simulink model "Reference_Simulink_Model"  (R2024a)
settings: Solver=VariableStepAuto  StartTime=0.0  StopTime=2800  RelTol=1e-3
undefined symbols (not defined in the file or in its folder): Amplitude_Wave_Lake, Amplitude_Wind_Lake, Factor_Wave_1, Factor_Wave_2, Frequency_Wave_Lake, Frequency_Wind_Lake, Gain_Derivative_Controller, Gain_Integral_Controller, Gain_Proportional_Controller, Gain_Wind, Position_Initial_X, Position_Initial_Y, Static_Gain_Waves, Time_Constant_Wind, Velocity_Ship_Mean, Waypoints
libraries: cstblocks x2, simulink x2
settings Model: Creator=gerar  LastModifiedBy=gerar

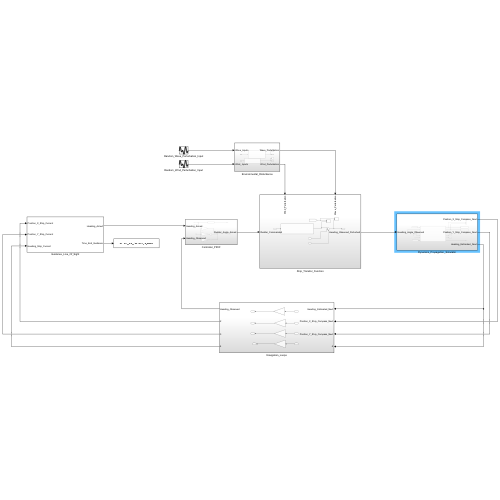
[thumbnail: Simulink's stored preview of the top-level diagram]
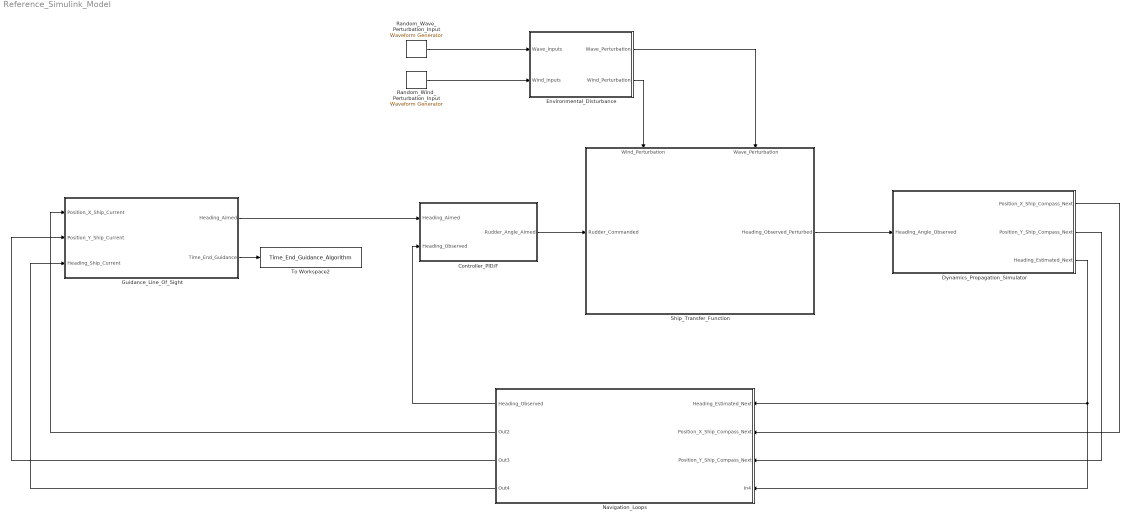
== system Reference_Simulink_Model ==
  Controller_PID/F : Subsystem
  Dynamics_Propagation_Simulator : Subsystem
  Environmental_Disturbance : Subsystem
  Guidance_Line_Of_Sight : Subsystem
  Navigation_Loops : Subsystem
  Random_Wave_Perturbation_Input : simulink/Sources/Waveform Generator  OutMin=[]  OutMax=[]  OutDataTypeStr=double  SelectedSignal=1  Signals=sin(Amplitude_Wave_Lake, Frequency_Wave_Lake, 1)  BlockNames=MultiportSwitch_4566f8e7d9dc4b1  SampleTime=0.1
  Random_Wind_Perturbation_Input : simulink/Sources/Waveform Generator  OutMin=[]  OutMax=[]  OutDataTypeStr=double  SelectedSignal=1  Signals=sin(Amplitude_Wind_Lake, Frequency_Wind_Lake, 1)  BlockNames=MultiportSwitch_bec1be775c304e8  SampleTime=0.1
  Ship_Transfer_Function : Subsystem
      settings: PortSchema="{\"entries\":[{\"content\":{\"sides\":[{\"content\":{\"connectorIds\":[\"In1\"]},\"type\":\"ConnectorPlacement.EquallySpacedRectSide\",\"uuid\":\"39a47681-8a87-4f22-9e16-0ead526089e0\"},{\"content\":{\"connectorIds\":[\"Out1\"],\"side\":\"RIGHT\"},\"type\":\"ConnectorPlacement.EquallySpacedRectSide\",\"uuid\":\"e7d068dc-643f-44db-a553-0a54b66f6b70\"},{\"content\":{\"connectorIds\":[\"In2\",\"In3\"],\"side\":\"TOP\"},\"type\":\"ConnectorPlacement.EquallySpacedRectSide\",\"uuid\":\"f984f23d-1b96-40dd-a354-9bced51babaa\"}]},\"type\":\"ConnectorPlacement.EquallySpacedConnector\",\"uuid\":\"30082198-c592-4bfc-a5f8-ae0235b1924b\"}],\"packageUris\":[\"http://schema.mathworks.com/mf0/Connector/R2020b\"],\"version\":\"1.0\"}"
  To Workspace2 : ToWorkspace  VariableName=Time_End_Guidance_Algorithm  SaveFormat=Timeseries  SampleTime=-1
  wires:
  Guidance_Line_Of_Sight/1(Heading_Aimed) -> Controller_PID/F/1(Heading_Aimed)
  Controller_PID/F/1(Rudder_Angle_Aimed) -> Ship_Transfer_Function/1(Rudder_Commanded)
  Guidance_Line_Of_Sight/2(Time_End_Guidance) -> To Workspace2/1
  Random_Wave_Perturbation_Input/1 -> Environmental_Disturbance/1(Wave_Inputs)
  Random_Wind_Perturbation_Input/1 -> Environmental_Disturbance/2(Wind_Inputs)
  Environmental_Disturbance/1(Wave_Perturbation) -> Ship_Transfer_Function/3(Wave_Perturbation)
  Environmental_Disturbance/2(Wind_Perturbation) -> Ship_Transfer_Function/2(Wind_Perturbation)
  Navigation_Loops/1(Heading_Observed) -> Controller_PID/F/2(Heading_Observed)
  Ship_Transfer_Function/1(Heading_Observed_Perturbed) -> Dynamics_Propagation_Simulator/1(Heading_Angle_Observed)
  Dynamics_Propagation_Simulator/3(Heading_Estimated_Next) -> Navigation_Loops/4(In4), Navigation_Loops/1(Heading_Estimated_Next)
  Dynamics_Propagation_Simulator/1(Position_X_Ship_Compass_Next) -> Navigation_Loops/2(Position_X_Ship_Compass_Next)
  Navigation_Loops/2(Out2) -> Guidance_Line_Of_Sight/1(Position_X_Ship_Current)
  Dynamics_Propagation_Simulator/2(Position_Y_Ship_Compass_Next) -> Navigation_Loops/3(Position_Y_Ship_Compass_Next)
  Navigation_Loops/3(Out3) -> Guidance_Line_Of_Sight/2(Position_Y_Ship_Current)
  Navigation_Loops/4(Out4) -> Guidance_Line_Of_Sight/3(Heading_Ship_Current)

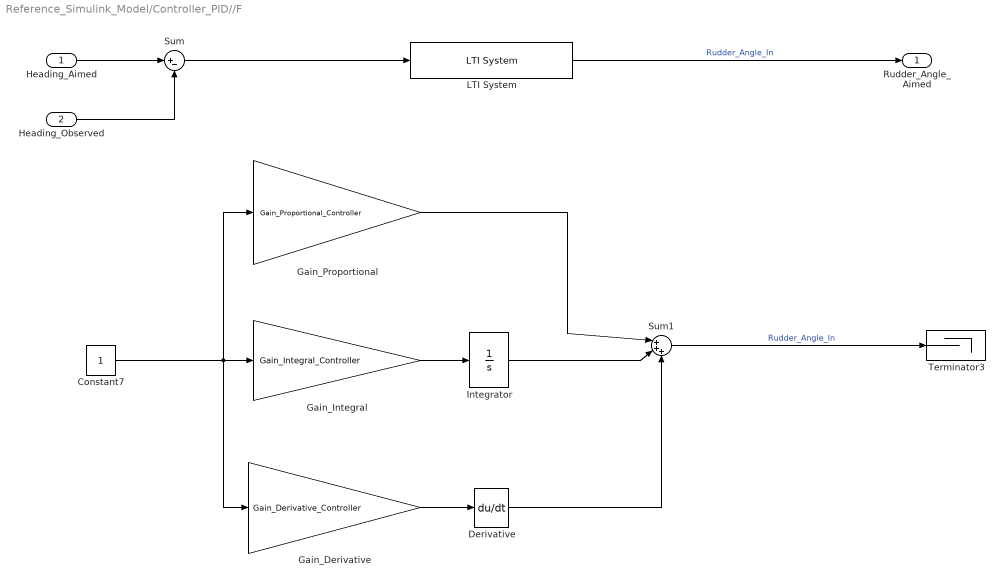
== system Reference_Simulink_Model/Controller_PID//F ==
  Heading_Aimed : Inport
  Heading_Observed : Inport  Port=2
  Constant7 : Constant
  Derivative : Derivative
  Gain_Derivative : Gain  Gain=Gain_Derivative_Controller
  Gain_Integral : Gain  Gain=Gain_Integral_Controller
  Gain_Proportional : Gain  Gain=Gain_Proportional_Controller
  Integrator : Integrator
  LTI System : cstblocks/LTI System  sys=Controller_PIDF  IC=[]  PadeOrder=0
  Sum : Sum  Inputs=|+-
  Sum1 : Sum  Inputs=|+++
  Terminator3 : Terminator
  Rudder_Angle_Aimed : Outport
  wires:
  Heading_Aimed/1 -> Sum/1
  Heading_Observed/1 -> Sum/2
  Sum1/1 -> Terminator3/1  "Rudder_Angle_In"
  Gain_Proportional/1 -> Sum1/1
  Integrator/1 -> Sum1/2
  Gain_Integral/1 -> Integrator/1
  Constant7/1 -> Gain_Proportional/1, Gain_Integral/1, Gain_Derivative/1
  Gain_Derivative/1 -> Derivative/1
  Derivative/1 -> Sum1/3
  Sum/1 -> LTI System/1
  LTI System/1 -> Rudder_Angle_Aimed/1  "Rudder_Angle_In"

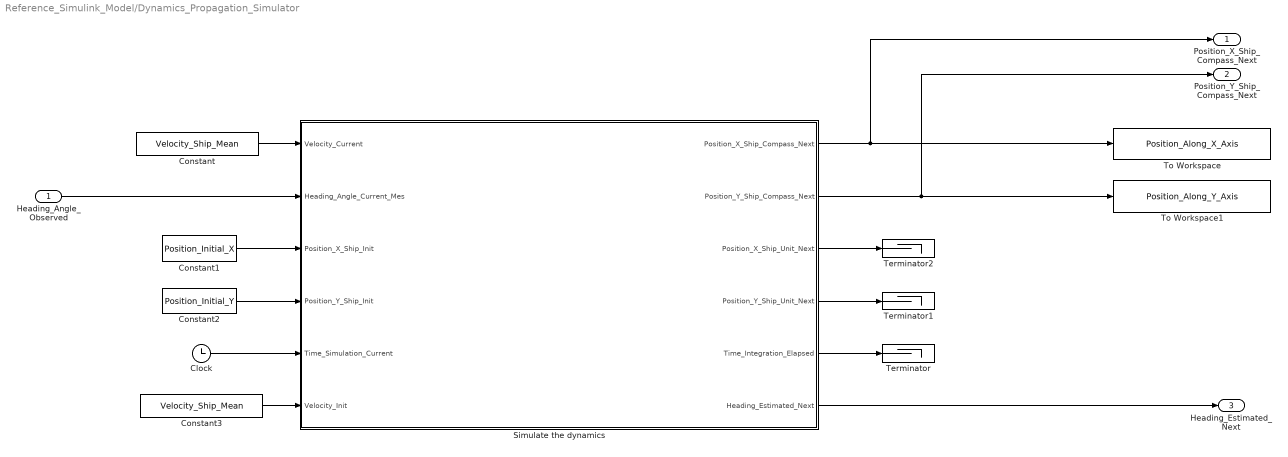
== system Reference_Simulink_Model/Dynamics_Propagation_Simulator ==
  Heading_Angle_Observed : Inport
  Clock : Clock
  Constant : Constant  Value=Velocity_Ship_Mean
  Constant1 : Constant  Value=Position_Initial_X
  Constant2 : Constant  Value=Position_Initial_Y
  Constant3 : Constant  Value=Velocity_Ship_Mean
  Simulate the dynamics : MATLAB Function  TreatAsAtomicUnit=on
  Terminator : Terminator
  Terminator1 : Terminator
  Terminator2 : Terminator
  To Workspace : ToWorkspace  VariableName=Position_Along_X_Axis  SaveFormat=Timeseries  SampleTime=-1
  To Workspace1 : ToWorkspace  VariableName=Position_Along_Y_Axis  SaveFormat=Timeseries  SampleTime=-1
  Position_X_Ship_Compass_Next : Outport
  Position_Y_Ship_Compass_Next : Outport  Port=2
  Heading_Estimated_Next : Outport  Port=3
  wires:
  Simulate the dynamics/1(Position_X_Ship_Compass_Next) -> Position_X_Ship_Compass_Next/1, To Workspace/1
  Heading_Angle_Observed/1 -> Simulate the dynamics/2(Heading_Angle_Current_Mes)
  Simulate the dynamics/5(Time_Integration_Elapsed) -> Terminator/1
  Simulate the dynamics/4(Position_Y_Ship_Unit_Next) -> Terminator1/1
  Constant1/1 -> Simulate the dynamics/3(Position_X_Ship_Init)
  Constant/1 -> Simulate the dynamics/1(Velocity_Current)
  Simulate the dynamics/2(Position_Y_Ship_Compass_Next) -> Position_Y_Ship_Compass_Next/1, To Workspace1/1
  Simulate the dynamics/3(Position_X_Ship_Unit_Next) -> Terminator2/1
  Constant2/1 -> Simulate the dynamics/4(Position_Y_Ship_Init)
  Clock/1 -> Simulate the dynamics/5(Time_Simulation_Current)
  Simulate the dynamics/6(Heading_Estimated_Next) -> Heading_Estimated_Next/1
  Constant3/1 -> Simulate the dynamics/6(Velocity_Init)

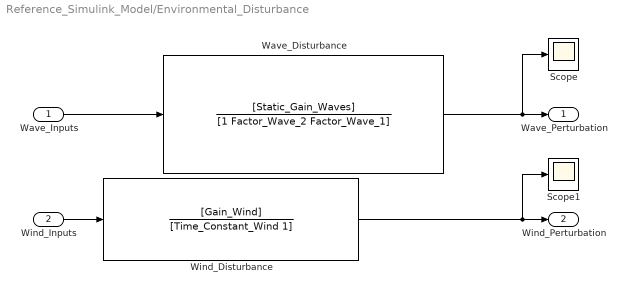
== system Reference_Simulink_Model/Environmental_Disturbance ==
  Wave_Inputs : Inport
  Wind_Inputs : Inport  Port=2
  Scope : Scope
  Scope1 : Scope
  Wave_Disturbance : TransferFcn  Numerator=[Static_Gain_Waves]  Denominator=[1 Factor_Wave_2 Factor_Wave_1]
  Wind_Disturbance : TransferFcn  Numerator=[Gain_Wind]  Denominator=[Time_Constant_Wind 1]
  Wave_Perturbation : Outport
  Wind_Perturbation : Outport  Port=2
  wires:
  Wind_Inputs/1 -> Wind_Disturbance/1
  Wave_Disturbance/1 -> Scope/1, Wave_Perturbation/1
  Wave_Inputs/1 -> Wave_Disturbance/1
  Wind_Disturbance/1 -> Scope1/1, Wind_Perturbation/1

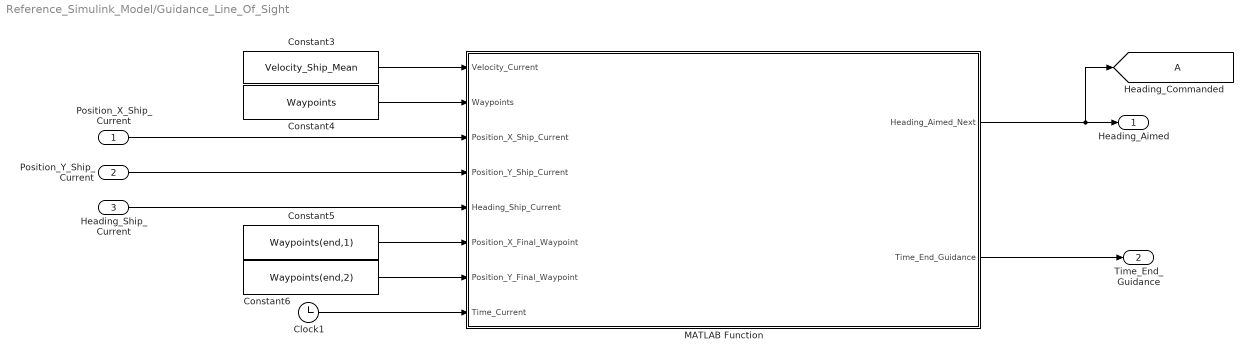
== system Reference_Simulink_Model/Guidance_Line_Of_Sight ==
  Position_X_Ship_Current : Inport
  Position_Y_Ship_Current : Inport  Port=2
  Heading_Ship_Current : Inport  Port=3
  Clock1 : Clock
  Constant3 : Constant  Value=Velocity_Ship_Mean
  Constant4 : Constant  Value=Waypoints
  Constant5 : Constant  Value=Waypoints(end,1)
  Constant6 : Constant  Value=Waypoints(end,2)
  Heading_Commanded : Goto  TagVisibility=global
  MATLAB Function : MATLAB Function  TreatAsAtomicUnit=on
  Heading_Aimed : Outport
  Time_End_Guidance : Outport  Port=2
  wires:
  Constant5/1 -> MATLAB Function/6(Position_X_Final_Waypoint)
  Position_X_Ship_Current/1 -> MATLAB Function/3(Position_X_Ship_Current)
  MATLAB Function/1(Heading_Aimed_Next) -> Heading_Commanded/1, Heading_Aimed/1
  Constant4/1 -> MATLAB Function/2(Waypoints)
  Constant3/1 -> MATLAB Function/1(Velocity_Current)
  Constant6/1 -> MATLAB Function/7(Position_Y_Final_Waypoint)
  Clock1/1 -> MATLAB Function/8(Time_Current)
  Position_Y_Ship_Current/1 -> MATLAB Function/4(Position_Y_Ship_Current)
  MATLAB Function/2(Time_End_Guidance) -> Time_End_Guidance/1
  Heading_Ship_Current/1 -> MATLAB Function/5(Heading_Ship_Current)

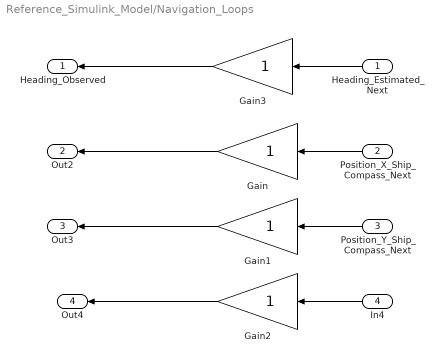
== system Reference_Simulink_Model/Navigation_Loops ==
  Heading_Estimated_Next : Inport
  Position_X_Ship_Compass_Next : Inport  Port=2
  Position_Y_Ship_Compass_Next : Inport  Port=3
  In4 : Inport  Port=4
  Gain{,1..3} (4 alike) : Gain
  Heading_Observed : Outport
  Out2 : Outport  Port=2
  Out3 : Outport  Port=3
  Out4 : Outport  Port=4
  wires:
  Heading_Estimated_Next/1 -> Gain3/1
  Gain1/1 -> Out3/1
  In4/1 -> Gain2/1
  Gain2/1 -> Out4/1
  Position_X_Ship_Compass_Next/1 -> Gain/1
  Gain/1 -> Out2/1
  Position_Y_Ship_Compass_Next/1 -> Gain1/1
  Gain3/1 -> Heading_Observed/1

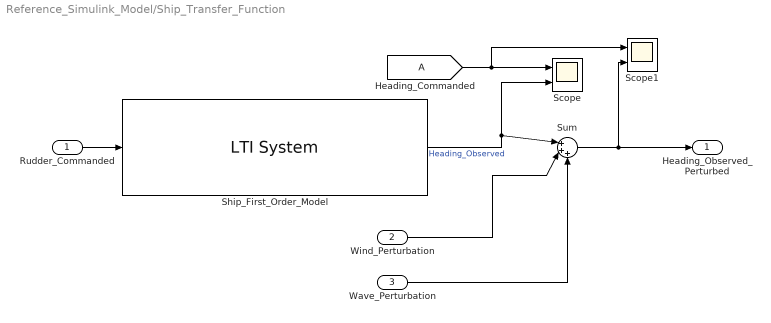
== system Reference_Simulink_Model/Ship_Transfer_Function ==
  Rudder_Commanded : Inport
  Wind_Perturbation : Inport  Port=2
  Wave_Perturbation : Inport  Port=3
  Heading_Commanded : From  TagVisibility=global
  Scope : Scope  NumInputPorts=2
  Scope1 : Scope  NumInputPorts=2
  Ship_First_Order_Model : cstblocks/LTI System  sys=Heading_On_Rudder_Transfer_First_Order  IC=[]  PadeOrder=0
  Sum : Sum  Inputs=|+++
  Heading_Observed_Perturbed : Outport
  wires:
  Ship_First_Order_Model/1 -> Sum/1, Scope/2  "Heading_Observed"
  Rudder_Commanded/1 -> Ship_First_Order_Model/1
  Heading_Commanded/1 -> Scope1/1, Scope/1
  Sum/1 -> Scope1/2, Heading_Observed_Perturbed/1
  Wind_Perturbation/1 -> Sum/2
  Wave_Perturbation/1 -> Sum/3

== matlab function Reference_Simulink_Model/Guidance_Line_Of_Sight/MATLAB Function ==
  settings: updateMethod=DISCRETE
  data: Velocity_Current input; Heading_Aimed_Next output; Waypoints input; Position_X_Ship_Current input; Position_Y_Ship_Current input; Heading_Ship_Current input; Position_X_Final_Waypoint input; Position_Y_Final_Waypoint input; Time_Current input; Time_End_Guidance output
function [Heading_Aimed_Next,Time_End_Guidance] = Guidance_Waypoints_Following(Velocity_Current,...
                                                                               Waypoints,...
                                                                               Position_X_Ship_Current,...
                                                                               Position_Y_Ship_Current,...
                                                                               Heading_Ship_Current,...
                                                                               Position_X_Final_Waypoint,...
                                                                               Position_Y_Final_Waypoint,...
                                                                               Time_Current)

% Terminal point features:
Position_X_Final_Point = Position_X_Final_Waypoint;
Position_Y_Final_Point = Position_Y_Final_Waypoint;
Radius_Final_Waypoint = 50;

% Enable Guidance to work if the ship is not close to the final waypoint:
if ~((Position_X_Ship_Current - Position_X_Final_Point)^2 + (Position_Y_Ship_Current - Position_Y_Final_Point)^2 <= Radius_Final_Waypoint^2)

    % Then settle the time of end Guidance:
    Time_End_Guidance = 0;

    % Retreive the aimed heading angle that must be performed at this step time
    % of the simulation to follow the Waypoints generated trajectory:
    [Heading_Aimed_Unit,Heading_Aimed_Compass,...
     Heading_Error_Unit,Heading_Error_Compass,...
     Selected_Waypoints,Heading_Current_Unit] = Guidance_Heading_Rudder_Angle(Waypoints,...
                                                                              Position_X_Ship_Current,...
                                                                              Position_Y_Ship_Current, ...
                                                                              Heading_Ship_Current);

else
    
    [Heading_Aimed_Unit,Heading_Aimed_Compass,...
     Heading_Error_Unit,Heading_Error_Compass,...
     Selected_Waypoints,Heading_Current_Unit] = Guidance_Heading_Rudder_Angle(Waypoints,...
                                                                              Position_X_Ship_Current,...
                                                                              Position_Y_Ship_Current, ...
                                                                              Heading_Ship_Current);

    % Then determine the end time of the Guidance scheme:
    Time_End_Guidance = Time_Current;

end

% Then order the heading aimed:
Heading_Aimed_Next = Heading_Aimed_Compass;

end

== matlab function Reference_Simulink_Model/Dynamics_Propagation_Simulator/Simulate the dynamics ==
  settings: updateMethod=DISCRETE
  data: Velocity_Current input; Position_X_Ship_Compass_Next output; Heading_Angle_Current_Mes input; Position_X_Ship_Init input; Position_Y_Ship_Init input; Time_Simulation_Current input; Position_Y_Ship_Compass_Next output; Position_X_Ship_Unit_Next output; Position_Y_Ship_Unit_Next output; Time_Integration_Elapsed output; Heading_Estimated_Next output; Velocity_Init input
function [Position_X_Ship_Compass_Next,Position_Y_Ship_Compass_Next,...
          Position_X_Ship_Unit_Next,Position_Y_Ship_Unit_Next,...
          Time_Integration_Elapsed,Heading_Estimated_Next] = Dynamics_Propagation(Velocity_Current,Heading_Angle_Current_Mes,...
                                                                                  Position_X_Ship_Init,Position_Y_Ship_Init,...
                                                                                  Time_Simulation_Current,Velocity_Init)

% Persistents definition:
persistent Position_X_Ship_Compass_Prev
persistent Position_Y_Ship_Compass_Prev
persistent Position_X_Ship_Unit_Prev
persistent Position_Y_Ship_Unit_Prev
persistent Time_Simulation_Previous

% See if the measured heading angle needs conversion to unit circle:
Heading_Angle_Current_Mes_Unit = -Heading_Angle_Current_Mes + (pi/2);

% Simulation time handeling persistent:
if isempty(Time_Simulation_Previous)
    Time_Simulation_Previous = Time_Simulation_Current;
    Time_Integration_Elapsed = Time_Simulation_Current - Time_Simulation_Previous;
else
    Time_Integration_Elapsed = Time_Simulation_Current - Time_Simulation_Previous;
end
Time_Simulation_Previous = Time_Simulation_Current;

% Calculate the local position increment but use both convention (unit and compass):
% Compass:
Position_X_Ship_Current_Increment_Compass = Time_Integration_Elapsed*Velocity_Current*sin(Heading_Angle_Current_Mes);
Position_Y_Ship_Current_Increment_Compass = Time_Integration_Elapsed*Velocity_Current*cos(Heading_Angle_Current_Mes);
% Unit:
Position_X_Ship_Current_Increment_Unit = Time_Integration_Elapsed*Velocity_Current*cos(Heading_Angle_Current_Mes_Unit);
Position_Y_Ship_Current_Increment_Unit = Time_Integration_Elapsed*Velocity_Current*sin(Heading_Angle_Current_Mes_Unit);

% Compass position persistent filling:
if isempty(Position_X_Ship_Compass_Prev)
    Position_X_Ship_Compass_Prev = Position_X_Ship_Init + Position_X_Ship_Current_Increment_Compass;
else
    Position_X_Ship_Compass_Prev = Position_X_Ship_Compass_Prev + Position_X_Ship_Current_Increment_Compass;
end
if isempty(Position_Y_Ship_Compass_Prev)
    Position_Y_Ship_Compass_Prev = Position_Y_Ship_Init + Position_Y_Ship_Current_Increment_Compass;
else
    Position_Y_Ship_Compass_Prev = Position_Y_Ship_Compass_Prev + Position_Y_Ship_Current_Increment_Compass;
end
% Unit position persistent filling:
if isempty(Position_X_Ship_Unit_Prev)
    Position_X_Ship_Unit_Prev = Position_X_Ship_Init + Position_X_Ship_Current_Increment_Unit;
else
    Position_X_Ship_Unit_Prev = Position_X_Ship_Unit_Prev + Position_X_Ship_Current_Increment_Unit;
end
if isempty(Position_Y_Ship_Unit_Prev)
    Position_Y_Ship_Unit_Prev = Position_Y_Ship_Init + Position_Y_Ship_Current_Increment_Unit;
else
    Position_Y_Ship_Unit_Prev = Position_Y_Ship_Unit_Prev + Position_Y_Ship_Current_Increment_Unit;
end


% Then update the persistents:
% Compass:
Position_X_Ship_Compass_Next = Position_X_Ship_Compass_Prev;
Position_Y_Ship_Compass_Next = Position_Y_Ship_Compass_Prev;
% Unit:
Position_X_Ship_Unit_Next = Position_X_Ship_Unit_Prev;
Position_Y_Ship_Unit_Next = Position_Y_Ship_Unit_Prev;

% Just propagate the estimated heading:
Heading_Estimated_Next = Heading_Angle_Current_Mes;

end
